simulink model "ksp_zad12"  (Simulink 2.20)
settings: Solver=ode45  StartTime=0.0  StopTime=20  RelTol=1e-3  AbsTol=1e-6
settings Model: ConsistencyChecking=off  RTWPlaceOutputsASAP=off

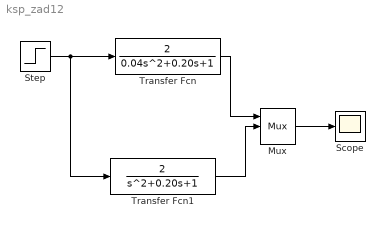
== system ksp_zad12 ==
  Mux : Mux  Inputs=3
  Scope : Scope
      settings: TickLabels=on  TimeRange=20  YMin=-0.5  YMax=4  SaveToWorkspace=off  SaveName=ScopeData
  Step : Step  Time=1  Before=0  After=1
  Transfer Fcn : TransferFcn  Numerator=[2]  Denominator=[0.04 0.20 1]
  Transfer Fcn1 : TransferFcn  Numerator=[2]  Denominator=[1 0.20 1]
  wires:
  Transfer Fcn/1 -> Mux/1
  Mux/1 -> Scope/1
  Step/1 -> Transfer Fcn1/1, Transfer Fcn/1
  Transfer Fcn1/1 -> Mux/2
